simulink model "Seven_Mathematical_Modelling_of_DC_Motor"  (R2024a)
settings: Solver=ode23tb  StartTime=0.0  StopTime=10.0  MaxStep=1e-4  RelTol=1e-3
settings Model: Creator=91889  LastModifiedBy=91889

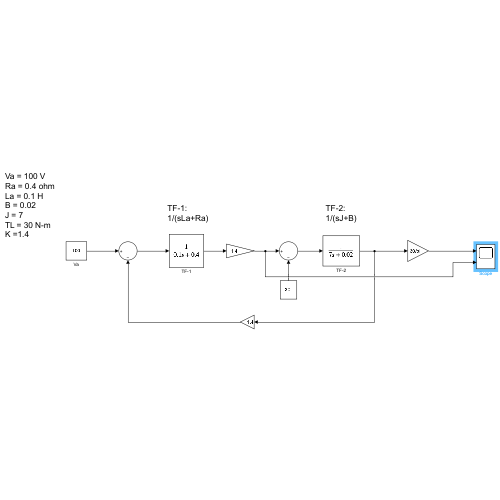
[thumbnail: Simulink's stored preview of the top-level diagram]
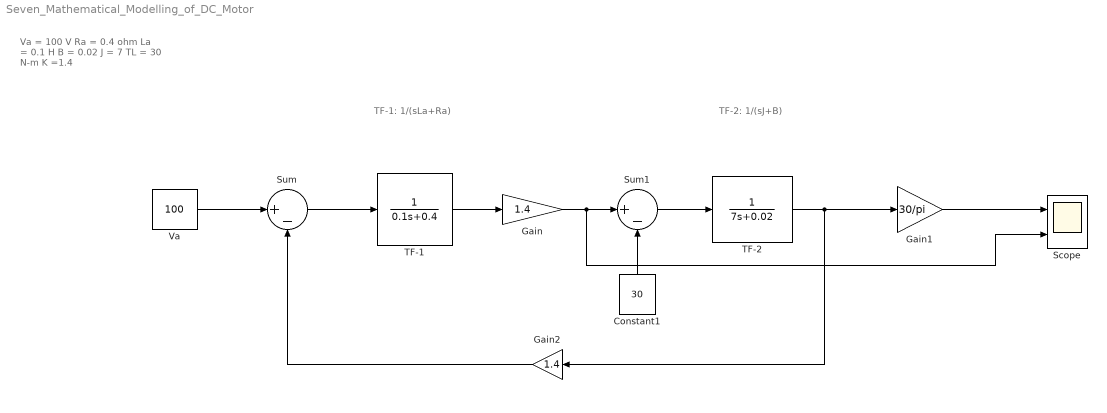
== system Seven_Mathematical_Modelling_of_DC_Motor ==
  note: TF-1:
      | 1/(sLa+Ra)
  note: Va = 100 V
      | Ra = 0.4 ohm
      | La = 0.1 H
      | B = 0.02
      | J = 7
      | TL = 30 N-m
      | K =1.4
  note: TF-2:
      | 1/(sJ+B)
  Constant1 : Constant  Value=30
  Gain : Gain  Gain=1.4
  Gain1 : Gain  Gain=30/pi
  Gain2 : Gain  Gain=1.4
  Scope : Scope  NumInputPorts=2
  Sum : Sum  Inputs=|+-
  Sum1 : Sum  Inputs=|+-
  TF-1 : TransferFcn  Denominator=[0.1 0.4]
  TF-2 : TransferFcn  Denominator=[7 0.02]
  Va : Constant  Value=100
  wires:
  Va/1 -> Sum/1
  Sum/1 -> TF-1/1
  TF-1/1 -> Gain/1
  Gain/1 -> Scope/2, Sum1/1
  Sum1/1 -> TF-2/1
  TF-2/1 -> Gain2/1, Gain1/1
  Gain1/1 -> Scope/1
  Constant1/1 -> Sum1/2
  Gain2/1 -> Sum/2
